simulink model "boom_to_imu_angles"  (R2016b)
settings: configuration reference "Configuration1khz" (kept outside this file)
values from neighbouring files (symbols this model uses):
  sample_time = 0.0005    [ElmoIncremental.m]
libraries: simulink x1
settings Model: xpc_rtwmakecfg_data=_xpcethercatlib_  SimulationMode=external  Creator=wmartin  LastModifiedBy=Will
settings ConfigSetRef: SourceLocation=Base Workspace

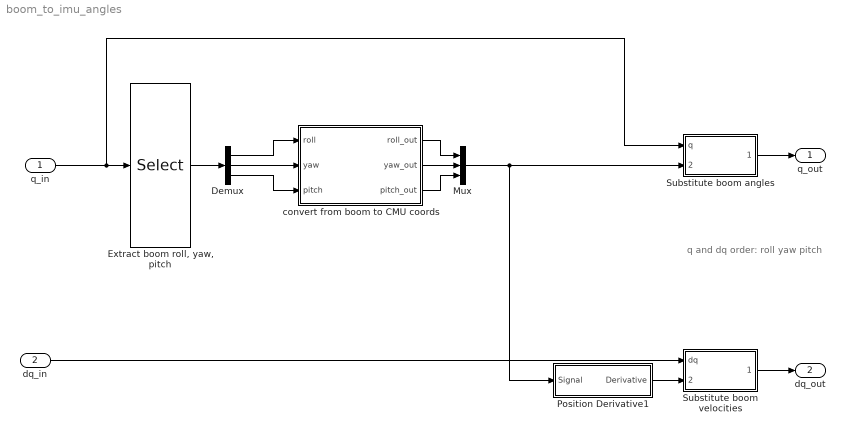
== system boom_to_imu_angles ==
  note: q and dq order:
      | 	roll
      | 	yaw
      | 	pitch
  q_in : Inport
  dq_in : Inport  Port=2
  Demux : Demux  Outputs=3
  "Extract boom roll, yaw, pitch" : Selector  InputPortWidth=13  IndexOptions=Index vector (dialog)  Indices=[11 12 13]  OutputSizes=1
  Mux : Mux  Inputs=3
  Position Derivative1 : Subsystem
  Substitute boom angles : Subsystem
  Substitute boom velocities : Subsystem
  convert from boom to CMU coords : MATLAB Function  TreatAsAtomicUnit=on
  q_out : Outport
  dq_out : Outport  Port=2
  wires:
  Substitute boom angles/1(Substituted) -> q_out/1
  q_in/1 -> Substitute boom angles/1(q), "Extract boom roll, yaw, pitch"/1
  "Extract boom roll, yaw, pitch"/1 -> Demux/1
  Demux/1 -> convert from boom to CMU coords/1(roll)
  Demux/2 -> convert from boom to CMU coords/2(yaw)
  Demux/3 -> convert from boom to CMU coords/3(pitch)
  convert from boom to CMU coords/2(yaw_out) -> Mux/2
  convert from boom to CMU coords/1(roll_out) -> Mux/1
  convert from boom to CMU coords/3(pitch_out) -> Mux/3
  Mux/1 -> Substitute boom angles/2(CMU Coords), Position Derivative1/1(Signal)
  dq_in/1 -> Substitute boom velocities/1(dq)
  Substitute boom velocities/1(Substituted) -> dq_out/1
  Position Derivative1/1(Derivative) -> Substitute boom velocities/2(CMU Coords)

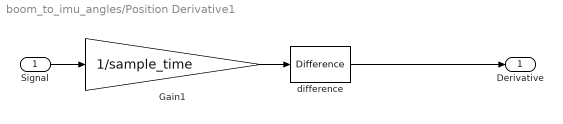
== system boom_to_imu_angles/Position Derivative1 ==
  Signal : Inport  SampleTime=sample_time
  Gain1 : Gain  Gain=1/sample_time
  difference : simulink/Discrete/Difference  ICPrevInput=0.0  InputProcessing=Inherited  OutMin=[]  OutMax=[]  OutDataType=fixdt(1, 16)  OutScaling=2^-10  DoSatur=off
  Derivative : Outport  SampleTime=sample_time
  wires:
  Gain1/1 -> difference/1
  Signal/1 -> Gain1/1
  difference/1 -> Derivative/1

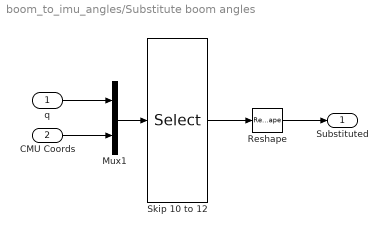
== system boom_to_imu_angles/Substitute boom angles ==
  q : Inport
  CMU Coords : Inport  Port=2
  Mux1 : Mux  Inputs=2
  Reshape : Reshape
  Skip 10 to 12 : Selector  InputPortWidth=16  IndexOptions=Index vector (dialog)  Indices=[1 2 3 4 5 6 7 8 9 10 14 15 16]  OutputSizes=1
  Substituted : Outport
  wires:
  CMU Coords/1 -> Mux1/2
  q/1 -> Mux1/1
  Skip 10 to 12/1 -> Reshape/1
  Mux1/1 -> Skip 10 to 12/1
  Reshape/1 -> Substituted/1

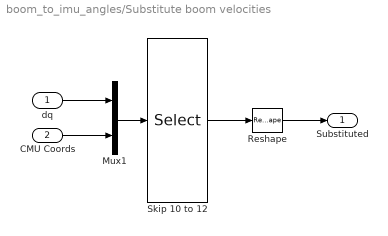
== system boom_to_imu_angles/Substitute boom velocities ==
  dq : Inport
  CMU Coords : Inport  Port=2
  Mux1 : Mux  Inputs=2
  Reshape : Reshape
  Skip 10 to 12 : Selector  InputPortWidth=16  IndexOptions=Index vector (dialog)  Indices=[1 2 3 4 5 6 7 8 9 10 14 15 16]  OutputSizes=1
  Substituted : Outport
  wires:
  Reshape/1 -> Substituted/1
  Mux1/1 -> Skip 10 to 12/1
  Skip 10 to 12/1 -> Reshape/1
  dq/1 -> Mux1/1
  CMU Coords/1 -> Mux1/2

== matlab function boom_to_imu_angles/convert from boom to CMU coords ==
  data: roll input; yaw input; pitch input; roll_out output; yaw_out output; pitch_out output
function [roll_out, yaw_out, pitch_out] = world2body(roll, yaw, pitch)

    % Generate rotation matrix from world to body frame
    roll = roll - 7.2824*pi/180;
    pitch = -pitch;
    R_yaw_world = [cos(yaw), -sin(yaw), 0; sin(yaw), cos(yaw), 0; 0, 0, 1];
    R_roll_world = [1, 0, 0; 0, cos(roll), -sin(roll); 0, sin(roll), cos(roll)];
    R_pitch_world = [cos(pitch), 0, sin(pitch); 0, 1, 0; -sin(pitch), 0, cos(pitch)];
    R_world2body = R_pitch_world*R_roll_world*R_yaw_world;

    % Extract euler angles
    yaw_out = atan2( R_world2body(2,1), R_world2body(1,1) );
    pitch_out  = atan2(-R_world2body(3,1), sqrt(R_world2body(3,2)^2+R_world2body(3,3)^2));
    roll_out   = atan2( R_world2body(3,2), R_world2body(3,3));
    
end
